simulink model "E33_VCU_simulink"  (R2014a)
settings: Solver=FixedStepDiscrete  StartTime=0.0  StopTime=10.0  FixedStep=0.0005  RelTol=1e-3
values from neighbouring files (symbols this model uses):
  Accu_FAN_Test = ecucoder_cal(Accu_FAN_Test)    [E33_VCU.m]
  Accu_FAN_threshold = ecucoder_cal(Accu_FAN_threshold)    [E33_VCU.m]
  APPS1_Voltage = ecucoder_cal(APPS1_Voltage)    [E33_VCU.m]
  APPS2_Voltage = ecucoder_cal(APPS2_Voltage)    [E33_VCU.m]
  APPS_Map = [0,1000]    [E33_VCU.m]
  APPS_threshold = ecucoder_cal(APPS_threshold)    [E33_VCU.m]
  Beep_Time = ecucoder_cal(Beep_Time)    [E33_VCU.m]
  BeeperTest = ecucoder_cal(BeeperTest)    [E33_VCU.m]
  BMSLedTest = ecucoder_cal(BMSLedTest)    [E33_VCU.m]
  BP_F_threshold = ecucoder_cal(BP_F_threshold)    [E33_VCU.m]
  BP_F_Voltage = ecucoder_cal(BP_F_Voltage)    [E33_VCU.m]
  BP_Map = [0,1000]    [E33_VCU.m]
  BP_R_Voltage = ecucoder_cal(BP_R_Voltage)    [E33_VCU.m]
  Brk_luminance = ecucoder_cal(Brk_luminance)    [E33_VCU.m]
  DCDC_Relay_Test = ecucoder_cal(DCDC_Relay_Test)    [E33_VCU.m]
  FactoryTestEnable = ecucoder_cal(FactoryTestEnable)    [E33_VCU.m]
  HardBrk_luminance = ecucoder_cal(HardBrk_luminance)    [E33_VCU.m]
  IMDLedTest = ecucoder_cal(IMDLedTest)    [E33_VCU.m]
  linear_FL_Map = ecucoder_cal(linear_FL_Map)    [E33_VCU.m]
  linear_FR_Map = ecucoder_cal(linear_FR_Map)    [E33_VCU.m]
  linear_Map = ecucoder_cal(linear_Map)    [E33_VCU.m]
  linear_RL_Map = ecucoder_cal(linear_RL_Map)    [E33_VCU.m]
  linear_RR_Map = ecucoder_cal(linear_RR_Map)    [E33_VCU.m]
  MaxPow = 40    [E33_VCU.m]
  MaxRPM = 5400    [E33_VCU.m]
  MaxRPMchangePerSec = ecucoder_cal(MaxRPMchangePerSec)    [E33_VCU.m]
  MaxTorqChangePerSec = ecucoder_cal(MaxTorqChangePerSec)    [E33_VCU.m]
  Motor_RPM_Map = (0:ceil(MaxRPM/100))*100    [E33_VCU.m]
  Pump_Test = ecucoder_cal(Pump_Test)    [E33_VCU.m]
  Pump_threshold = ecucoder_cal(Pump_threshold)    [E33_VCU.m]
  R2D_Light_Test = ecucoder_cal(R2D_Light_Test)    [E33_VCU.m]
  Radiator_FAN_Test = ecucoder_cal(Radiator_FAN_Test)    [E33_VCU.m]
  SCS_Error_5V = ecucoder_cal(SCS_Error_5V)    [E33_VCU.m]
  SCS_Error_GND = ecucoder_cal(SCS_Error_GND)    [E33_VCU.m]
  SPD_Coef = 1884/40    (= 47.1)    [E33_VCU.m]
  Tail_Light_Test = ecucoder_cal(Tail_Light_Test)    [E33_VCU.m]
  Tmanage_Map = [0,100]    [E33_VCU.m]
  Torq_percentage_Map = Motor_Torq_MAP/MaxTorq*1000    [E33_VCU.m]
libraries: simulink x164, ec55xxlib x44, dspswit3 x6
(part 1 of 5)
settings Model: Creator=lenovo  LastModifiedBy=lenovo
settings OptimizationCC: InlineParams=on  InlineInvariantSignals=on  RollThreshold=18  StateBitsets=on  DataBitsets=on  UseTempVars=on  ZeroExternalMemoryAtStartup=off  ZeroInternalMemoryAtStartup=off  EfficientFloat2IntCast=on  OptimizeModelRefInitCode=on  LifeSpan=1
settings DebuggingCC: InheritedTsInSrcMsg=none
settings HardwareCC: ProdLargestAtomicInteger=Long  ProdLargestAtomicFloat=Double  ProdIntDivRoundTo=Zero  ProdEndianess=BigEndian  ProdHWDeviceType=Freescale MPC5500
settings RTWCC: SystemTargetFile=ec55xx.tlc  MakeCommand=make_rtw optimized_fixed_point=1  GenerateMakefile=off  TemplateMakefile=ec55xx_lcc.tmf  PostCodeGenCommand=ec55xx_pst_s2(buildInfo)  Description=Target for EC55XX  GenerateReport=on  ProcessScript=ec55xx_make_rtw_hook  IncludeHyperlinkInReport=on  LaunchReport=on
settings CodeAppCC: IgnoreCustomStorageClasses=off
settings STFCustomTargetCC: ModelReferenceCompliant=off  ConcurrentExecutionCompliant=off  IncludeMdlTerminateFcn=off  GeneratePreprocessorConditionals=Use local settings  CombineOutputUpdateFcns=on  SuppressErrorStatus=on  ERTCustomFileBanners=on  SupportContinuousTime=off  SupportNonInlinedSFcns=off  MATLABClassNameForMDSCustomization=Simulink.SoftwareTarget.ERTCustomization  GRTInterface=off  SystemTargetFile=ec55xx.tlc
settings ERTTargetCC: GenerateSampleERTMain=off  ModelReferenceCompliant=off  IncludeMdlTerminateFcn=off  SuppressErrorStatus=on  GenerateASAP2=on  ERTSrcFileBannerTemplate=ec55xx_code_template.cgt  ERTHdrFileBannerTemplate=ec55xx_code_template.cgt  ERTDataSrcFileTemplate=ec55xx_code_template.cgt  ERTDataHdrFileTemplate=ec55xx_code_template.cgt  ERTCustomFileTemplate=ec55xx_file_process.tlc

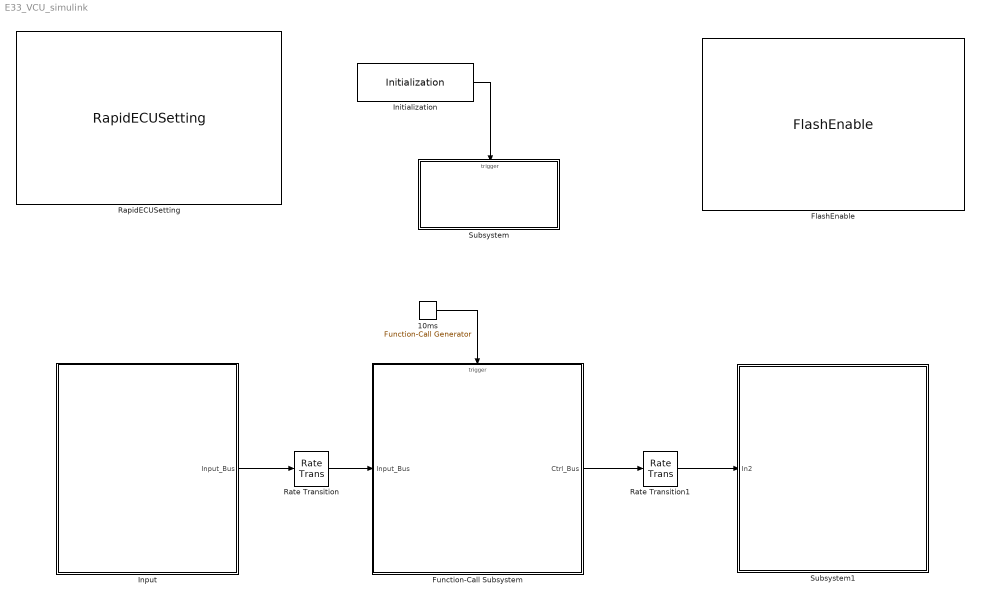
== system E33_VCU_simulink ==
  10ms : simulink/Ports & Subsystems/Function-Call Generator  sample_time=0.010  numberOfIterations=1
  FlashEnable : ec55xxlib/RapidECU_U2/10FlashManagement/FlashEnable  flashenable=on
  Function-Call Subsystem : Subsystem
  Initialization : ec55xxlib/RapidECU_U2/08MCUManagement/Initialization
  Input : Subsystem
  RapidECUSetting : ec55xxlib/RapidECU_U2/RapidECUSetting
      link override CAN: acmt=Extended(29-bit ID)  bcmt=Extended(29-bit ID)  apdf=1
      link override RTI: rtiperiod=0.0005
  Rate Transition : RateTransition
  Rate Transition1 : RateTransition
  Subsystem : Subsystem
  Subsystem1 : Subsystem
  wires:
  Initialization/1 -> Subsystem/Trigger
  Input/1(Input_Bus) -> Rate Transition/1
  Rate Transition/1 -> Function-Call Subsystem/1(Input_Bus)
  10ms/1 -> Function-Call Subsystem/Trigger
  Function-Call Subsystem/1(Ctrl_Bus) -> Rate Transition1/1
  Rate Transition1/1 -> Subsystem1/1(In2)

== system E33_VCU_simulink/Function-Call Subsystem ==
  Input_Bus : Inport
  function : TriggerPort  TriggerType=function-call
  Bus Creator : BusCreator  Inputs=2
  Bus Creator1 : BusCreator
  R2D_State : Subsystem
  Signal Conversion : SignalConversion
  Unit Delay : UnitDelay  SampleTime=-1
  Veh_Dynamic : Subsystem
  Warn : Subsystem
  Ctrl_Bus : Outport
  wires:
  Input_Bus/1 -> Bus Creator1/4, Bus Creator/2  "Input_Bus"
  Bus Creator1/1 -> Signal Conversion/1, Unit Delay/1  "Ctrl_Bus"
  Unit Delay/1 -> Bus Creator/1  "Ctrl_Bus_Delayed"
  Signal Conversion/1 -> Ctrl_Bus/1
  Bus Creator/1 -> R2D_State/1(In), Veh_Dynamic/1(Input_Bus), Warn/1(Warn_Msg)
  R2D_State/1(Out1) -> Bus Creator1/3  "R2D_State"
  Warn/1(Warn_level) -> Bus Creator1/1  "Warn"
  Veh_Dynamic/1(Out1) -> Bus Creator1/2  "Veh_Dynamic"

== system E33_VCU_simulink/Input ==
  Bus Creator : BusCreator  Inputs=6
  Input : Subsystem
  Input_Bus : Outport
  wires:
  Input/1("APP_Bus ") -> Bus Creator/1  "APP_Bus"
  Input/2("BP_Bus ") -> Bus Creator/2  "BP_Bus"
  Bus Creator/1 -> Input_Bus/1
  Input/3("Key_Bus ") -> Bus Creator/3  "Key_Bus"
  Input/4(Sensor_Bus) -> Bus Creator/4  "Sensor_Bus"
  Input/5(BMS_Bus) -> Bus Creator/5  "BMS_Bus"
  Input/6(MCU_Bus) -> Bus Creator/6  "MCU_Bus"

== system E33_VCU_simulink/Subsystem ==
  function : TriggerPort  TriggerType=function-call
  AfterRunSwitch : ec55xxlib/RapidECU_U2/09PowerManagement/AfterRunSwitch  sampletime=-1
  Constant : Constant  OutDataTypeStr=boolean
  PowerDriverSwitch : ec55xxlib/RapidECU_U2/04PowerDriverSwitch/PowerDriverSwitch  channel=99: O_MR_LS0A7  sampletime=-1
  wires:
  Constant/1 -> AfterRunSwitch/1, PowerDriverSwitch/1

== system E33_VCU_simulink/Subsystem1 ==
  In2 : Inport
  20ms : simulink/Ports & Subsystems/Function-Call Generator  sample_time=0.02  numberOfIterations=1
  20ms1 : simulink/Ports & Subsystems/Function-Call Generator  sample_time=0.02  numberOfIterations=1
  50ms{,1..3} (4 alike) : simulink/Ports & Subsystems/Function-Call Generator  sample_time=0.05  numberOfIterations=1
  DCDC_Ctrl : Subsystem
  MCUctrl : Subsystem  TreatAsAtomicUnit=on
  PanelCtrl : Subsystem  TreatAsAtomicUnit=on
  Rate Transition{1..6} (6 alike) : RateTransition
  TailLight : Subsystem  TreatAsAtomicUnit=on
  TmanageCtrl : Subsystem  TreatAsAtomicUnit=on
  VCUCAN : Subsystem
  wires:
  Rate Transition3/1 -> MCUctrl/1(In1)
  Rate Transition2/1 -> PanelCtrl/1(In1)
  50ms/1 -> PanelCtrl/Trigger
  20ms/1 -> MCUctrl/Trigger
  Rate Transition4/1 -> TailLight/1(In1)
  50ms1/1 -> TmanageCtrl/Trigger
  Rate Transition5/1 -> TmanageCtrl/1(In1)
  20ms1/1 -> TailLight/Trigger
  Rate Transition1/1 -> DCDC_Ctrl/1(In1)
  50ms2/1 -> DCDC_Ctrl/Trigger
  In2/1 -> Rate Transition3/1, Rate Transition6/1, Rate Transition1/1, Rate Transition5/1, Rate Transition4/1, Rate Transition2/1
  Rate Transition6/1 -> VCUCAN/1(In1)
  50ms3/1 -> VCUCAN/Trigger

== system E33_VCU_simulink/Function-Call Subsystem/R2D_State ==
  In : Inport
  Bus Creator1 : BusCreator  Inputs=3
  Bus Selector : BusSelector  OutputSignals=Input_Bus.Key_Bus.R2D_SW,Input_Bus.APP_Bus.APPS_Pos,Input_Bus.BP_Bus.BP_F_Pos,Input_Bus.MCU_Bus.MCU_Online,Input_Bus.MCU_Bus.MCU_Stat.MCU_IsReady
  Chart : Stateflow chart  RequirementInfo="{}  %GIDa_9082d276_9a80_43b5_a65a_81b478704c00"  TreatAsAtomicUnit=on
  Compare To Constant : simulink/Logic and Bit Operations/Compare To Constant  relop=<=  const=APPS_threshold  OutDataTypeStr=boolean
  Compare To Constant1 : simulink/Logic and Bit Operations/Compare To Constant  relop=>=  const=BP_F_threshold  OutDataTypeStr=boolean
  Constant : Constant  Value=Beep_Time
  Data Type Conversion{,1..3} (4 alike) : DataTypeConversion  OutDataTypeStr=boolean  RndMeth=Nearest
  Logical Operator : Logic  AllPortsSameDT=off  OutDataTypeStr=boolean
  Out1 : Outport
  wires:
  In/1 -> Bus Selector/1
  Bus Selector/2 -> Compare To Constant/1  "<APPS_Pos>"
  Bus Selector/3 -> Compare To Constant1/1  "<BP_F_Pos>"
  Bus Selector/4 -> Data Type Conversion/1  "<MCU_Online>"
  Bus Selector/5 -> Data Type Conversion1/1  "<MCU_IsReady>"
  Compare To Constant1/1 -> Data Type Conversion3/1
  Compare To Constant/1 -> Data Type Conversion2/1
  Chart/3(VehReady) -> Bus Creator1/3  "VehReady"
  Chart/2(VehStandby) -> Bus Creator1/2  "VehStandby"
  Chart/1(BeeperStOut) -> Bus Creator1/1  "BeeperOut"
  Bus Creator1/1 -> Out1/1
  Data Type Conversion/1 -> Logical Operator/1
  Data Type Conversion1/1 -> Logical Operator/2
  Logical Operator/1 -> Chart/4(MCU_Ready)  "MCU_Ready"
  Data Type Conversion2/1 -> Chart/2(APPS_OK)  "APPS_OK"
  Data Type Conversion3/1 -> Chart/3(BP_F_OK)  "BP_F_OK"
  Constant/1 -> Chart/5(Beep_Time)
  Bus Selector/1 -> Chart/1(R2D_SW)  "<R2D_SW>"

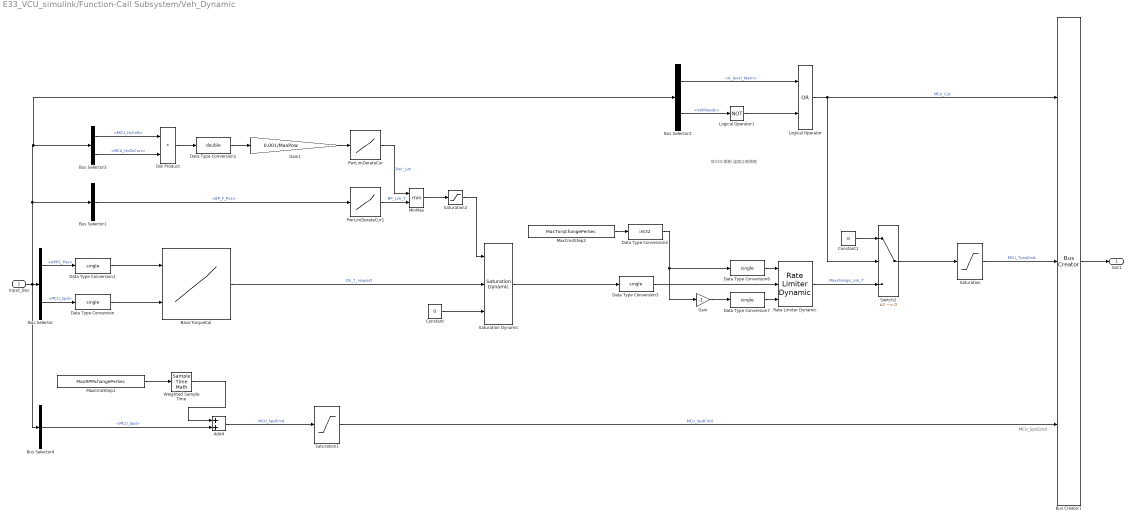
== system E33_VCU_simulink/Function-Call Subsystem/Veh_Dynamic ==
  note: 低SOC限制
      | 温度过高限制
  note: MCU_SpdCmd
  Input_Bus : Inport
  Add4 : Sum
  BasicTorqueCal : Lookup_n-D  BreakpointsForDimension1=[0,1000]  BreakpointsForDimension2=Motor_RPM_Map  Table=Torq_percentage_Map  TableDataTypeStr=Inherit: Inherit from 'Table data'  ExtrapMethod=Clip  InternalRulePriority=Speed  OutDataTypeStr=uint16  RndMeth=Simplest
  Bus Creator1 : BusCreator  Inputs=3
  Bus Selector : BusSelector  OutputSignals=Input_Bus.APP_Bus.APPS_Pos,Input_Bus.MCU_Bus.MCU_Stat.MCU_Spd
  Bus Selector1 : BusSelector  OutputSignals=Input_Bus.BP_Bus.BP_F_Pos
  Bus Selector2 : BusSelector  OutputSignals=Ctrl_Bus_Delayed.Warn.A_level_Warn,Ctrl_Bus_Delayed.R2D_State.VehReady
  Bus Selector3 : BusSelector  OutputSignals=Input_Bus.MCU_Bus.MCU_Power.MCU_HvVolt,Input_Bus.MCU_Bus.MCU_Power.MCU_HvDcCurr
  Bus Selector4 : BusSelector  OutputSignals=Input_Bus.MCU_Bus.MCU_Stat.MCU_Spd
  Constant : Constant  Value=0
  Constant1 : Constant  Value=0  OutDataTypeStr=uint16
  Data Type Conversion{,1,3,6..7} (5 alike) : DataTypeConversion  OutDataTypeStr=single
  Data Type Conversion2 : DataTypeConversion  OutDataTypeStr=double
  Data Type Conversion4 : DataTypeConversion  OutDataTypeStr=int32
  Dot Product : DotProduct  InputSameDT=on  OutDataTypeStr=Inherit: Inherit via internal rule
  Gain : Gain  Gain=-1
  Gain1 : Gain  Gain=0.001/MaxPow  OutDataTypeStr=single
  Logical Operator : Logic  Operator=OR  AllPortsSameDT=off  OutDataTypeStr=boolean
  Logical Operator1 : Logic  Operator=NOT  AllPortsSameDT=off  OutDataTypeStr=boolean
  MaxCmdStep1 : Constant  Value=MaxRPMchangePerSec  OutDataTypeStr=uint16
  MaxCmdStep2 : Constant  Value=MaxTorqChangePerSec  OutDataTypeStr=uint16
  MinMax : MinMax  Inputs=2
  PwrLimDerateCur : Lookup_n-D  NumberOfTableDimensions=1  BreakpointsForDimension1=[0.95,0.98,0.99]  BreakpointsForDimension1DataTypeStr=double  Table=[1000,500,0]  TableDataTypeStr=double  ExtrapMethod=Clip  InternalRulePriority=Speed  OutDataTypeStr=single  RndMeth=Simplest  InputSameDT=on
  PwrLimDerateCur1 : Lookup_n-D  NumberOfTableDimensions=1  BreakpointsForDimension1=[0,1000]  Table=[1000,0]  ExtrapMethod=Clip  InternalRulePriority=Speed  OutDataTypeStr=uint16  RndMeth=Simplest  InputSameDT=on
  Rate Limiter Dynamic : simulink/Discontinuities/Rate Limiter Dynamic
  Saturation : Saturate  UpperLimit=1000  LowerLimit=0
  Saturation Dynamic : simulink/Discontinuities/Saturation Dynamic  OutMin=[]  OutMax=[]  OutDataTypeStr=Inherit: Same as second input  OutDataType=fixdt(1, 16)  OutScaling=2^-10  DoSatur=off
  Saturation1 : Saturate  UpperLimit=MaxRPM  LowerLimit=-MaxRPM
  Saturation2 : Saturate  UpperLimit=1000  LowerLimit=0
  Switch2 : Switch  Criteria=u2 ~= 0
  Weighted Sample Time : SampleTimeMath  TsampMathOp=*
  Out1 : Outport
  wires:
  Input_Bus/1 -> Bus Selector4/1, Bus Selector2/1, Bus Selector3/1, Bus Selector1/1, Bus Selector/1
  Data Type Conversion/1 -> BasicTorqueCal/2
  Data Type Conversion1/1 -> BasicTorqueCal/1
  Bus Selector/1 -> Data Type Conversion1/1  "<APPS_Pos>"
  Bus Selector/2 -> Data Type Conversion/1  "<MCU_Spd>"
  Bus Selector1/1 -> PwrLimDerateCur1/1  "<BP_F_Pos>"
  Gain1/1 -> PwrLimDerateCur/1
  PwrLimDerateCur1/1 -> MinMax/2  "BP_Lim_T"
  PwrLimDerateCur/1 -> MinMax/1  "Pwr_Lim"
  MinMax/1 -> Saturation2/1
  Saturation2/1 -> Saturation Dynamic/1
  Dot Product/1 -> Data Type Conversion2/1
  Data Type Conversion2/1 -> Gain1/1
  Bus Selector3/1 -> Dot Product/1  "<MCU_HvVolt>"
  Bus Selector3/2 -> Dot Product/2  "<MCU_HvDcCurr>"
  BasicTorqueCal/1 -> Saturation Dynamic/2  "Dri_T_request"
  Constant/1 -> Saturation Dynamic/3
  Data Type Conversion4/1 -> Gain/1, Data Type Conversion6/1
  MaxCmdStep2/1 -> Data Type Conversion4/1
  Gain/1 -> Data Type Conversion7/1
  Data Type Conversion6/1 -> Rate Limiter Dynamic/1
  Data Type Conversion7/1 -> Rate Limiter Dynamic/3
  Data Type Conversion3/1 -> Rate Limiter Dynamic/2
  Logical Operator/1 -> Switch2/2, Bus Creator1/1  "MCU_Cut"
  Constant1/1 -> Switch2/1
  Saturation Dynamic/1 -> Data Type Conversion3/1
  Rate Limiter Dynamic/1 -> Switch2/3  "Maxchange_Lim_T"
  Switch2/1 -> Saturation/1
  Bus Selector4/1 -> Add4/2  "<MCU_Spd>"
  MaxCmdStep1/1 -> Weighted Sample Time/1
  Add4/1 -> Saturation1/1  "MCU_SpdCmd"
  Saturation/1 -> Bus Creator1/2  "MCU_TorqCmd"
  Saturation1/1 -> Bus Creator1/3  "MCU_SpdCmd"
  Bus Creator1/1 -> Out1/1
  Bus Selector2/1 -> Logical Operator/1  "<A_level_Warn>"
  Bus Selector2/2 -> Logical Operator1/1  "<VehReady>"
  Logical Operator1/1 -> Logical Operator/2
  Weighted Sample Time/1 -> Add4/1

== system E33_VCU_simulink/Function-Call Subsystem/Warn ==
  note: A级故障切断扭矩输出
      | B级故障显示告警信号
  Warn_Msg : Inport
  A_level_Warn : Subsystem
  B_level_Warn : Subsystem
  Bus Creator : BusCreator  Inputs=2
  Warn_level : Outport
  wires:
  Warn_Msg/1 -> B_level_Warn/1(In1), A_level_Warn/1(In1)
  A_level_Warn/1(A_level_Warn) -> Bus Creator/1  "A_level_Warn"
  B_level_Warn/1(B_level_Warn) -> Bus Creator/2  "B_level_Warn"
  Bus Creator/1 -> Warn_level/1

== system E33_VCU_simulink/Input/Input ==
  100ms : simulink/Ports & Subsystems/Function-Call Generator  sample_time=0.1  numberOfIterations=1
  10ms{,1..4} (5 alike) : simulink/Ports & Subsystems/Function-Call Generator  sample_time=0.010  numberOfIterations=1
  50ms : simulink/Ports & Subsystems/Function-Call Generator  sample_time=0.050  numberOfIterations=1
  APPS : Subsystem
  BMS_CAN_Receive : Subsystem  TreatAsAtomicUnit=on
  Bpressure : Subsystem
  Bus Creator : BusCreator
  Bus Creator1 : BusCreator
  Bus Creator2 : BusCreator  Inputs=1
  Bus Creator3 : BusCreator  Inputs=5
  Bus Creator4 : BusCreator  Inputs=5
  Bus Creator5 : BusCreator  Inputs=3
  Keys : Subsystem
  MCU_CAN_Receive : Subsystem
  Self_inspection : Subsystem
  Sensor : Subsystem
  "APP_Bus " : Outport
  "BP_Bus " : Outport  Port=2
  "Key_Bus " : Outport  Port=3
  Sensor_Bus : Outport  Port=4
  BMS_Bus : Outport  Port=5
  MCU_Bus : Outport  Port=6
  wires:
  10ms/1 -> APPS/Trigger
  10ms1/1 -> Bpressure/Trigger
  APPS/2(APPS_Unreliable) -> Bus Creator/2  "APPS_Unreliable"
  APPS/1(APPS_Pos) -> Bus Creator/1  "APPS_Pos"
  Bus Creator/1 -> "APP_Bus "/1
  Bus Creator1/1 -> "BP_Bus "/1
  50ms/1 -> Self_inspection/Trigger
  Bus Creator2/1 -> "Key_Bus "/1
  Keys/1(R2D_SW) -> Bus Creator2/1  "R2D_SW"
  10ms2/1 -> Keys/Trigger
  10ms3/1 -> Sensor/Trigger
  Sensor/1(Linear_RR) -> Bus Creator3/1  "Linear_RR"
  Sensor/3(Linear_RL) -> Bus Creator3/3  "Linear_RL"
  Sensor/2(Linear_FR) -> Bus Creator3/2  "Linear_FR"
  Sensor/4(Linear_FL) -> Bus Creator3/4  "Linear_FL"
  Sensor/5(Wheel_Angle) -> Bus Creator3/5  "Wheel_Angle"
  Bus Creator3/1 -> Sensor_Bus/1
  10ms4/1 -> MCU_CAN_Receive/Trigger
  100ms/1 -> BMS_CAN_Receive/Trigger
  BMS_CAN_Receive/2(BMS_INFO) -> Bus Creator4/2  "BMS_Info"
  Bus Creator4/1 -> BMS_Bus/1
  BMS_CAN_Receive/1(BMS_Online) -> Bus Creator4/1  "BMS_Online"
  BMS_CAN_Receive/3(BMS_ALM) -> Bus Creator4/3  "BMS_Alarm"
  BMS_CAN_Receive/4(BMS_MAXT) -> Bus Creator4/4  "BMS_MAXT"
  MCU_CAN_Receive/3(MCU_Power) -> Bus Creator5/3  "MCU_Power"
  MCU_CAN_Receive/2(MCU_Stat) -> Bus Creator5/2  "MCU_Stat"
  MCU_CAN_Receive/1(MCU_Online) -> Bus Creator5/1  "MCU_Online"
  Bus Creator5/1 -> MCU_Bus/1
  BMS_CAN_Receive/5(BMS_MAXV) -> Bus Creator4/5  "BMS_MAXV"
  APPS/3(APPS1_Disconnect) -> Bus Creator/3  "APPS1_Disconnect"
  APPS/4(APPS2_Disconnect) -> Bus Creator/4  "APPS2_Disconnect"
  Bpressure/3(BP_F_Disconnect) -> Bus Creator1/3  "BP_F_Disconnect"
  Bpressure/4(BP_R_Disconnect) -> Bus Creator1/4  "BP_R_Disconnect"
  Bpressure/1(BP_F_Pos) -> Bus Creator1/1  "BP_F_Pos"
  Bpressure/2(BP_R_Pos) -> Bus Creator1/2  "BP_R_Pos"

== system E33_VCU_simulink/Subsystem1/DCDC_Ctrl ==
  In1 : Inport
  function : TriggerPort  TriggerType=function-call
  Bus Selector3 : BusSelector  OutputSignals=Input_Bus.BMS_Bus.BMS_Info.BMS_Stat,Input_Bus.BMS_Bus.BMS_Online
  Compare To Constant1 : simulink/Logic and Bit Operations/Compare To Constant  relop===  const=5  OutDataTypeStr=boolean
  Constant4 : Constant  Value=FactoryTestEnable  OutDataTypeStr=Inherit: Inherit via back propagation
  Constant5 : Constant  Value=DCDC_Relay_Test  OutDataTypeStr=Inherit: Inherit via back propagation
  DCDC_Ctrl : Stateflow chart  TreatAsAtomicUnit=on
  DCDC_MR_CTRL : ec55xxlib/RapidECU_U2/04PowerDriverSwitch/PowerDriverSwitch  channel=60: O_PWM3_LS1A8  sampletime=-1
  Data Type Conversion3 : DataTypeConversion  OutDataTypeStr=boolean
  Logical Operator1 : Logic  AllPortsSameDT=off  OutDataTypeStr=boolean
  Switch1 : Switch  Criteria=u2 ~= 0
  wires:
  In1/1 -> Bus Selector3/1
  Logical Operator1/1 -> DCDC_Ctrl/1(HV_ON)
  Bus Selector3/2 -> Logical Operator1/2  "<BMS_Online>"
  Data Type Conversion3/1 -> Switch1/3  "DCDC_ON"
  Bus Selector3/1 -> Compare To Constant1/1  "<BMS_Stat>"
  Compare To Constant1/1 -> Logical Operator1/1
  Constant5/1 -> Switch1/1
  DCDC_Ctrl/1(DCDC_ON) -> Data Type Conversion3/1
  Switch1/1 -> DCDC_MR_CTRL/1  "DCDC_MR"
  Constant4/1 -> Switch1/2

== system E33_VCU_simulink/Subsystem1/MCUctrl ==
  In1 : Inport
  function : TriggerPort  TriggerType=function-call
  Bus Selector : BusSelector  OutputSignals=Veh_Dynamic.MCU_Cut,Veh_Dynamic.MCU_TorqCmd,Veh_Dynamic.MCU_SpdCmd
  Bus Selector1 : BusSelector  OutputSignals=Input_Bus.MCU_Bus.MCU_Online
  Constant : Constant
  Constant{1..5,8..9} (7 alike) : Constant  Value=0
  Constant10 : Constant
  Constant6 : Constant  Value=0  OutDataTypeStr=uint8
  Constant7 : Constant  Value=2
  Data Type Conversion{1..9} (9 alike) : DataTypeConversion  OutDataTypeStr=uint16
  Data Type Conversion10 : DataTypeConversion  OutDataTypeStr=int32
  Data Type Conversion11 : DataTypeConversion  OutDataTypeStr=int32
  In2 : InportShadow
  MCU_CMD_CAN_Tx : Subsystem  TreatAsAtomicUnit=on
  Switch1 : Switch  Criteria=u2 ~= 0
  Switch2 : Switch  Criteria=u2 ~= 0
  Terminator1 : Terminator
  VCU_MCU_CMD : Subsystem
  wires:
  In1/1 -> Bus Selector/1
  Constant/1 -> Data Type Conversion2/1
  Constant7/1 -> Switch1/3
  Constant1/1 -> Data Type Conversion5/1
  Constant2/1 -> Data Type Conversion6/1
  Constant3/1 -> Data Type Conversion7/1
  Constant4/1 -> Data Type Conversion9/1
  Switch2/1 -> Data Type Conversion8/1
  Bus Selector/2 -> Data Type Conversion10/1  "<MCU_TorqCmd>"
  Bus Selector/3 -> Data Type Conversion11/1  "<MCU_SpdCmd>"
  Bus Selector/1 -> Switch1/2, Switch2/2  "<MCU_Cut>"
  Constant6/1 -> Data Type Conversion1/1
  Data Type Conversion4/1 -> VCU_MCU_CMD/4(MCU_IsMcuNOTActive_in)
  Data Type Conversion1/1 -> VCU_MCU_CMD/1(MCU_HV_Voltage_in)
  Data Type Conversion2/1 -> VCU_MCU_CMD/2(MCU_IsPosRelayAct_in)
  Data Type Conversion3/1 -> VCU_MCU_CMD/3(MCU_GEAR_CMD_in)
  Data Type Conversion5/1 -> VCU_MCU_CMD/5(MCU_IsZeroLocMode_in)
  Data Type Conversion6/1 -> VCU_MCU_CMD/6(MCU_IsBrakeMode_in)
  Data Type Conversion7/1 -> VCU_MCU_CMD/7(MCU_IsSpdMode_in)
  Data Type Conversion8/1 -> VCU_MCU_CMD/8(MCU_IsTorqMode_in)
  Data Type Conversion9/1 -> VCU_MCU_CMD/9(MCU_IsFreeMode_in)
  Data Type Conversion10/1 -> VCU_MCU_CMD/10(MCU_TORQ_CMD_in)
  Data Type Conversion11/1 -> VCU_MCU_CMD/11(MCU_SPD_CMD_in)
  MCU_CMD_CAN_Tx/1(CAN_OK) -> Terminator1/1
  Switch1/1 -> Data Type Conversion3/1
  Constant8/1 -> Switch1/1
  Constant9/1 -> Data Type Conversion4/1
  Constant5/1 -> Switch2/1
  Constant10/1 -> Switch2/3
  VCU_MCU_CMD/1(output) -> MCU_CMD_CAN_Tx/1(Msg)
  In2/1 -> Bus Selector1/1
  Bus Selector1/1 -> MCU_CMD_CAN_Tx/Enable  "<MCU_Online>"

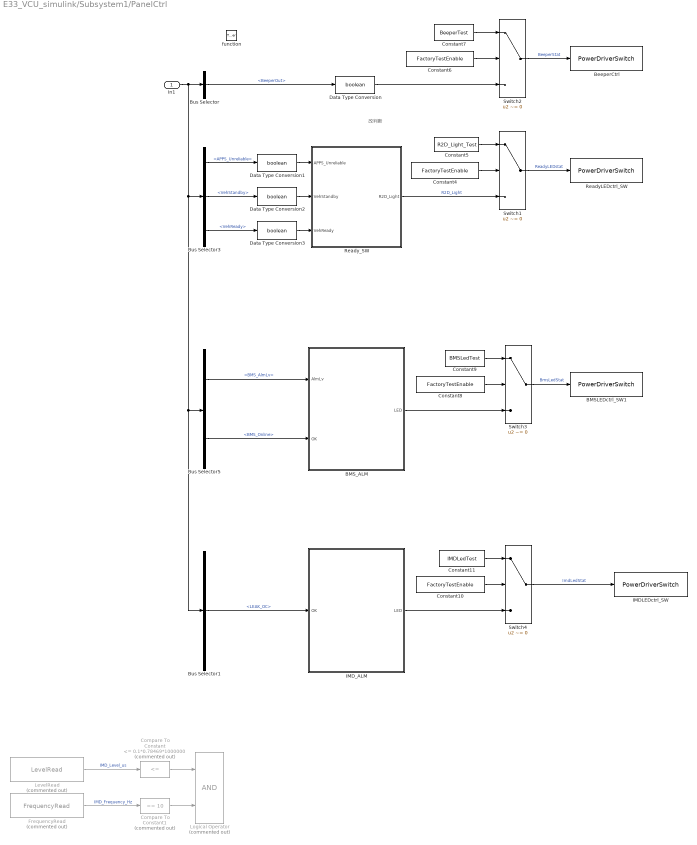
== system E33_VCU_simulink/Subsystem1/PanelCtrl ==
  note: 改判断
  In1 : Inport
  function : TriggerPort  TriggerType=function-call
  BMSLEDctrl_SW1 : ec55xxlib/RapidECU_U2/04PowerDriverSwitch/PowerDriverSwitch  channel=63: O_SW1_LS0A7  sampletime=-1
  BMS_ALM : Stateflow chart  TreatAsAtomicUnit=on
  BeeperCtrl : ec55xxlib/RapidECU_U2/04PowerDriverSwitch/PowerDriverSwitch  channel=79: O_SW3_LS0A7  sampletime=-1
  Bus Selector : BusSelector  OutputSignals=R2D_State.BeeperOut
  Bus Selector1 : BusSelector  OutputSignals=Input_Bus.BMS_Bus.BMS_Alarm.LEAK_OC
  Bus Selector3 : BusSelector  OutputSignals=Input_Bus.APP_Bus.APPS_Unreliable,R2D_State.VehStandby,R2D_State.VehReady
  Bus Selector5 : BusSelector  OutputSignals=Input_Bus.BMS_Bus.BMS_Info.BMS_AlmLv,Input_Bus.BMS_Bus.BMS_Online
  Compare To Constant : simulink/Logic and Bit Operations/Compare To Constant  Commented=on  relop=<=  const=0.1*0.78469*1000000  OutDataTypeStr=boolean
  Compare To Constant1 : simulink/Logic and Bit Operations/Compare To Constant  Commented=on  relop===  const=10  OutDataTypeStr=boolean
  Constant{4,6,8,10} (4 alike) : Constant  Value=FactoryTestEnable  OutDataTypeStr=Inherit: Inherit via back propagation
  Constant11 : Constant  Value=IMDLedTest  OutDataTypeStr=Inherit: Inherit via back propagation
  Constant5 : Constant  Value=R2D_Light_Test  OutDataTypeStr=Inherit: Inherit via back propagation
  Constant7 : Constant  Value=BeeperTest  OutDataTypeStr=Inherit: Inherit via back propagation
  Constant9 : Constant  Value=BMSLedTest  OutDataTypeStr=Inherit: Inherit via back propagation
  Data Type Conversion{,1..3} (4 alike) : DataTypeConversion  OutDataTypeStr=boolean
  FrequencyRead : ec55xxlib/RapidECU_U2/03FrequencyInput/FrequencyRead  Commented=on  channel=37: I_HALL1  sampletime=-1
  IMDLEDctrl_SW : ec55xxlib/RapidECU_U2/04PowerDriverSwitch/PowerDriverSwitch  channel=78: O_SW2_LS0A7  sampletime=-1
  IMD_ALM : Stateflow chart  TreatAsAtomicUnit=on
  LevelRead : ec55xxlib/RapidECU_U2/03FrequencyInput/LevelRead  Commented=on  channel=37: I_HALL1  activelevel=Active High  sampletime=-1
  Logical Operator : Logic  Commented=on  AllPortsSameDT=off  OutDataTypeStr=boolean
  ReadyLEDctrl_SW : ec55xxlib/RapidECU_U2/04PowerDriverSwitch/PowerDriverSwitch  channel=58: O_PWM1_LS1A8  sampletime=-1
  Ready_SW : Stateflow chart  TreatAsAtomicUnit=on
  Switch{1..4} (4 alike) : Switch  Criteria=u2 ~= 0
  wires:
  Bus Selector/1 -> Data Type Conversion/1  "<BeeperOut>"
  In1/1 -> Bus Selector1/1, Bus Selector5/1, Bus Selector3/1, Bus Selector/1
  Ready_SW/1(R2D_Light) -> Switch1/3  "R2D_Light"
  Constant4/1 -> Switch1/2
  Constant5/1 -> Switch1/1
  Switch1/1 -> ReadyLEDctrl_SW/1  "ReadyLEDstat"
  Data Type Conversion/1 -> Switch2/3
  Constant6/1 -> Switch2/2
  Constant7/1 -> Switch2/1
  Switch2/1 -> BeeperCtrl/1  "BeeperStat"
  BMS_ALM/1(LED) -> Switch3/3
  Constant8/1 -> Switch3/2
  Constant9/1 -> Switch3/1
  Switch3/1 -> BMSLEDctrl_SW1/1  "BmsLedStat"
  Constant10/1 -> Switch4/2
  Constant11/1 -> Switch4/1
  Bus Selector5/1 -> BMS_ALM/1(AlmLv)  "<BMS_AlmLv>"
  Bus Selector5/2 -> BMS_ALM/2(OK)  "<BMS_Online>"
  Bus Selector3/1 -> Data Type Conversion1/1  "<APPS_Unreliable>"
  Bus Selector3/2 -> Data Type Conversion2/1  "<VehStandby>"
  Bus Selector3/3 -> Data Type Conversion3/1  "<VehReady>"
  Data Type Conversion1/1 -> Ready_SW/1(APPS_Unreliable)
  Data Type Conversion2/1 -> Ready_SW/2(VehStandby)
  Data Type Conversion3/1 -> Ready_SW/3(VehReady)
  FrequencyRead/1 -> Compare To Constant1/1  "IMD_Frequency_Hz"
  LevelRead/1 -> Compare To Constant/1  "IMD_Level_us"
  Compare To Constant/1 -> Logical Operator/1
  Compare To Constant1/1 -> Logical Operator/2
  Bus Selector1/1 -> IMD_ALM/1(OK)  "<LEAK_OC>"
  IMD_ALM/1(LED) -> Switch4/3
  Switch4/1 -> IMDLEDctrl_SW/1  "ImdLedStat"

== system E33_VCU_simulink/Subsystem1/TailLight ==
  In1 : Inport
  function : TriggerPort  TriggerType=function-call
  Bus Selector1 : BusSelector  OutputSignals=Input_Bus.BP_Bus.BP_F_Pos
  Compare To Constant : simulink/Logic and Bit Operations/Compare To Constant  relop=>=  const=80  OutDataTypeStr=boolean
  Compare To Constant1 : simulink/Logic and Bit Operations/Compare To Constant  relop=>=  const=950  OutDataTypeStr=boolean
  Constant : Constant  Value=5000  OutDataTypeStr=uint32
  Constant1 : Constant  Value=Brk_luminance
  Constant2 : Constant  Value=HardBrk_luminance
  Constant5 : Constant  Value=Tail_Light_Test  OutDataTypeStr=uint32
  Constant8 : Constant  Value=FactoryTestEnable  OutDataTypeStr=Inherit: Inherit via back propagation
  Data Type Conversion1 : DataTypeConversion  OutDataTypeStr=uint32
  Gain : Gain  Gain=50
  LED : Stateflow chart  TreatAsAtomicUnit=on
  Switch1 : Switch  Criteria=u2 ~= 0
  TailLightctrl : ec55xxlib/RapidECU_U2/06PowerDriverPWM/PowerDriverPWM  channel=61: O_PWM4_LS1A8  sampletime=-1
  wires:
  Constant/1 -> TailLightctrl/1
  Data Type Conversion1/1 -> TailLightctrl/2  "TailLightOnTime"
  In1/1 -> Bus Selector1/1
  Gain/1 -> Data Type Conversion1/1
  LED/1(LEDDutyCyc) -> Switch1/3
  Switch1/1 -> Gain/1
  Bus Selector1/1 -> Compare To Constant1/1, Compare To Constant/1  "<BP_F_Pos>"
  Compare To Constant1/1 -> LED/2(IsHardBrk)
  Compare To Constant/1 -> LED/1(IsBrk)
  Constant5/1 -> Switch1/1
  Constant8/1 -> Switch1/2
  Constant1/1 -> LED/3(Brk_luminance)
  Constant2/1 -> LED/4(HardBrk_luminance)

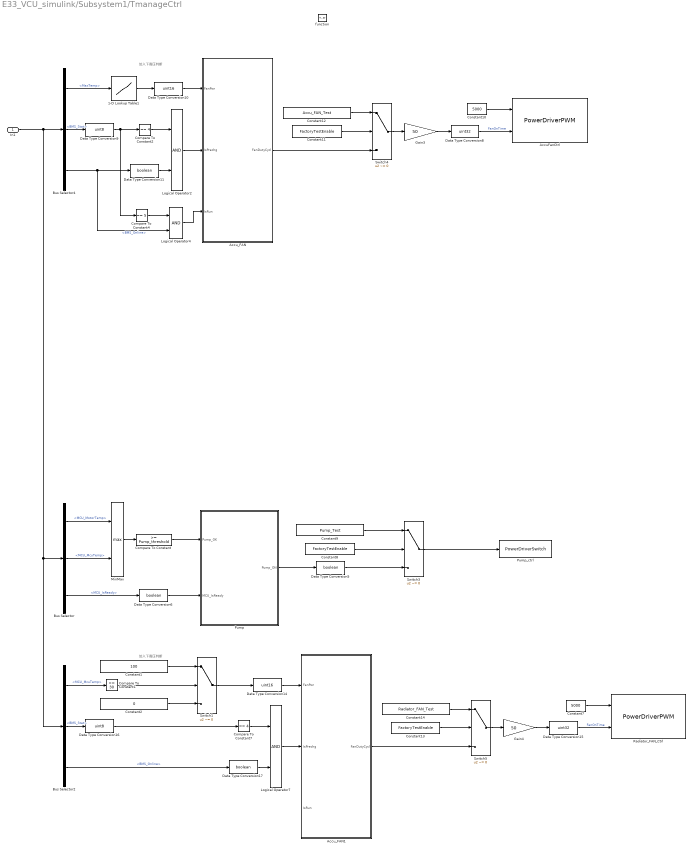
== system E33_VCU_simulink/Subsystem1/TmanageCtrl ==
  note: 加入下高压判断
  note: 加入下高压判断
  In1 : Inport
  function : TriggerPort  TriggerType=function-call
  1-D Lookup Table1 : Lookup_n-D  NumberOfTableDimensions=1  BreakpointsForDimension1=Accu_FAN_threshold  Table=Tmanage_Map  ExtrapMethod=Clip  InternalRulePriority=Speed  RndMeth=Simplest  InputSameDT=on
  AccuFanCtrl : ec55xxlib/RapidECU_U2/06PowerDriverPWM/PowerDriverPWM  channel=117: O_PWM11_HS2A9  sampletime=-1
  Accu_FAN : Stateflow chart  TreatAsAtomicUnit=on
  Accu_FAN1 : Stateflow chart  TreatAsAtomicUnit=on
  Bus Selector : BusSelector  OutputSignals=Input_Bus.MCU_Bus.MCU_Power.MCU_MotorTemp,Input_Bus.MCU_Bus.MCU_Power.MCU_McuTemp,Input_Bus.MCU_Bus.MCU_Stat.MCU_IsReady
  Bus Selector2 : BusSelector  OutputSignals=Input_Bus.MCU_Bus.MCU_Power.MCU_McuTemp,Input_Bus.BMS_Bus.BMS_Info.BMS_Stat,Input_Bus.BMS_Bus.BMS_Online
  Bus Selector4 : BusSelector  OutputSignals=Input_Bus.BMS_Bus.BMS_MAXT.MaxTemp,Input_Bus.BMS_Bus.BMS_Info.BMS_Stat,Input_Bus.BMS_Bus.BMS_Online
  Compare To Constant : simulink/Logic and Bit Operations/Compare To Constant  relop=>=  const=Pump_threshold  OutDataTypeStr=boolean
  Compare To Constant1 : simulink/Logic and Bit Operations/Compare To Constant  relop=>=  const=30  OutDataTypeStr=boolean
  Compare To Constant2 : simulink/Logic and Bit Operations/Compare To Constant  relop===  const=4  OutDataTypeStr=boolean
  Compare To Constant4 : simulink/Logic and Bit Operations/Compare To Constant  relop===  const=5  OutDataTypeStr=boolean
  Compare To Constant7 : simulink/Logic and Bit Operations/Compare To Constant  relop===  const=4  OutDataTypeStr=boolean
  Constant1 : Constant  Value=100  OutDataTypeStr=uint32
  Constant10 : Constant  Value=5000  OutDataTypeStr=uint32
  Constant11 : Constant  Value=FactoryTestEnable  OutDataTypeStr=Inherit: Inherit via back propagation
  Constant12 : Constant  Value=Accu_FAN_Test  OutDataTypeStr=uint32
  Constant13 : Constant  Value=FactoryTestEnable  OutDataTypeStr=Inherit: Inherit via back propagation
  Constant14 : Constant  Value=Radiator_FAN_Test  OutDataTypeStr=uint32
  Constant2 : Constant  Value=0  OutDataTypeStr=uint32
  Constant7 : Constant  Value=5000  OutDataTypeStr=uint32
  Constant8 : Constant  Value=FactoryTestEnable  OutDataTypeStr=Inherit: Inherit via back propagation
  Constant9 : Constant  Value=Pump_Test  OutDataTypeStr=Inherit: Inherit via back propagation
  Data Type Conversion10 : DataTypeConversion  OutDataTypeStr=uint16
  Data Type Conversion{5..6,11,17} (4 alike) : DataTypeConversion  OutDataTypeStr=boolean
  Data Type Conversion14 : DataTypeConversion  OutDataTypeStr=uint16
  Data Type Conversion15 : DataTypeConversion  OutDataTypeStr=uint32
  Data Type Conversion16 : DataTypeConversion  OutDataTypeStr=uint8
  Data Type Conversion8 : DataTypeConversion  OutDataTypeStr=uint32
  Data Type Conversion9 : DataTypeConversion  OutDataTypeStr=uint8
  Gain3 : Gain  Gain=50
  Gain4 : Gain  Gain=50
  Logical Operator2 : Logic  AllPortsSameDT=off  OutDataTypeStr=boolean
  Logical Operator4 : Logic  AllPortsSameDT=off  OutDataTypeStr=boolean
  Logical Operator7 : Logic  AllPortsSameDT=off  OutDataTypeStr=boolean
  MinMax : MinMax  Function=max  Inputs=2
  Pump : Stateflow chart  TreatAsAtomicUnit=on
  Pump_ctrl : ec55xxlib/RapidECU_U2/04PowerDriverSwitch/PowerDriverSwitch  channel=59: O_PWM2_LS1A8  sampletime=-1
  Radiator_FAN_Ctrl : ec55xxlib/RapidECU_U2/06PowerDriverPWM/PowerDriverPWM  channel=115: O_PWM10_HS2A9  sampletime=-1
  Switch{1,3..5} (4 alike) : Switch  Criteria=u2 ~= 0
  wires:
  Constant10/1 -> AccuFanCtrl/1
  Data Type Conversion8/1 -> AccuFanCtrl/2  "FanOnTime"
  Gain3/1 -> Data Type Conversion8/1
  Accu_FAN/1(FanDutyCycl) -> Switch4/3
  Constant11/1 -> Switch4/2
  Constant12/1 -> Switch4/1
  Switch4/1 -> Gain3/1
  Data Type Conversion9/1 -> Compare To Constant2/1, Compare To Constant4/1
  Compare To Constant2/1 -> Logical Operator2/1
  Bus Selector4/1 -> 1-D Lookup Table1/1  "<MaxTemp>"
  1-D Lookup Table1/1 -> Data Type Conversion10/1
  Data Type Conversion10/1 -> Accu_FAN/1(FanPwr)
  Logical Operator2/1 -> Accu_FAN/2(IsPrechg)
  Data Type Conversion11/1 -> Logical Operator2/2
  Bus Selector4/2 -> Data Type Conversion9/1  "<BMS_Stat>"
  Bus Selector4/3 -> Logical Operator4/2, Data Type Conversion11/1  "<BMS_Online>"
  Compare To Constant4/1 -> Logical Operator4/1
  Logical Operator4/1 -> Accu_FAN/3(IsRun)
  Constant7/1 -> Radiator_FAN_Ctrl/1
  Data Type Conversion15/1 -> Radiator_FAN_Ctrl/2  "FanOnTime"
  Gain4/1 -> Data Type Conversion15/1
  Accu_FAN1/1(FanDutyCycl) -> Switch5/3
  Constant13/1 -> Switch5/2
  Constant14/1 -> Switch5/1
  Switch5/1 -> Gain4/1
  Data Type Conversion16/1 -> Compare To Constant7/1
  Compare To Constant7/1 -> Logical Operator7/1
  Bus Selector2/1 -> Compare To Constant1/1  "<MCU_McuTemp>"
  Switch1/1 -> Data Type Conversion14/1
  Data Type Conversion14/1 -> Accu_FAN1/1(FanPwr)
  Logical Operator7/1 -> Accu_FAN1/2(IsPrechg)
  Data Type Conversion17/1 -> Logical Operator7/2
  Bus Selector2/2 -> Data Type Conversion16/1  "<BMS_Stat>"
  Bus Selector2/3 -> Data Type Conversion17/1  "<BMS_Online>"
  Constant8/1 -> Switch3/2
  Bus Selector/2 -> MinMax/2  "<MCU_McuTemp>"
  Bus Selector/1 -> MinMax/1  "<MCU_MotorTemp>"
  MinMax/1 -> Compare To Constant/1
  In1/1 -> Bus Selector/1, Bus Selector2/1, Bus Selector4/1
  Bus Selector/3 -> Data Type Conversion6/1  "<MCU_IsReady>"
  Compare To Constant/1 -> Pump/1(Pump_OK)
  Pump/1(Pump_ON) -> Data Type Conversion5/1
  Data Type Conversion5/1 -> Switch3/3
  Constant9/1 -> Switch3/1
  Data Type Conversion6/1 -> Pump/2(MCU_IsReady)
  Switch3/1 -> Pump_ctrl/1
  Constant1/1 -> Switch1/1
  Compare To Constant1/1 -> Switch1/2
  Constant2/1 -> Switch1/3

== system E33_VCU_simulink/Subsystem1/VCUCAN ==
  In1 : Inport
  function : TriggerPort  TriggerType=function-call
  Bus Selector3 : BusSelector  OutputSignals=Input_Bus.Sensor_Bus.Linear_RR,Input_Bus.Sensor_Bus.Linear_FR,Input_Bus.Sensor_Bus.Linear_RL,Input_Bus.Sensor_Bus.Linear_FL,Input_Bus.Sensor_Bus.Wheel_Angle
  CANTransmit : ec55xxlib/RapidECU_U2/07CANCommucation/CANTransmit  canmodule=A  canbuffer=8  canmessageid=hex2dec('17000000')  canmessagetype=Extended(29-bit ID)  datalength=8  sampletime=-1
  Terminator1 : Terminator
  VCU_Panel : Subsystem
  wires:
  In1/1 -> Bus Selector3/1
  CANTransmit/1 -> Terminator1/1
  Bus Selector3/1 -> VCU_Panel/2(Linear_RR_in)  "<Linear_RR>"
  Bus Selector3/2 -> VCU_Panel/3(Linear_FR_in)  "<Linear_FR>"
  Bus Selector3/3 -> VCU_Panel/4(Linear_RL_in)  "<Linear_RL>"
  Bus Selector3/4 -> VCU_Panel/5(Linear_FL_in)  "<Linear_FL>"
  Bus Selector3/5 -> VCU_Panel/1(Wheel_Angle_in)  "<Wheel_Angle>"
  VCU_Panel/1(output) -> CANTransmit/1

== system E33_VCU_simulink/Function-Call Subsystem/Warn/A_level_Warn ==
  In1 : Inport
  Bus Selector : BusSelector  OutputSignals=Input_Bus.MCU_Bus.MCU_Online,Input_Bus.APP_Bus.APPS_Unreliable,Input_Bus.APP_Bus.APPS1_Disconnect,Input_Bus.APP_Bus.APPS2_Disconnect,Input_Bus.BP_Bus.BP_F_Disconnect,Input_Bus.BP_Bus.BP_R_Disconnect
  Compare To Constant : simulink/Logic and Bit Operations/Compare To Constant  relop===  const=1  OutDataTypeStr=boolean
  Compare To Constant1 : simulink/Logic and Bit Operations/Compare To Constant  relop===  const=1  OutDataTypeStr=boolean
  Compare To Constant2 : simulink/Logic and Bit Operations/Compare To Constant  relop===  const=1  OutDataTypeStr=boolean
  Compare To Constant5 : simulink/Logic and Bit Operations/Compare To Constant  relop=~=  const=1  OutDataTypeStr=boolean
  Data Type Conversion{,1..2,5} (4 alike) : DataTypeConversion  OutDataTypeStr=boolean
  Logical Operator : Logic  Operator=OR  Inputs=1  IconShape=distinctive  AllPortsSameDT=off  OutDataTypeStr=boolean
  Mux : Mux  Inputs=6
  A_level_Warn : Outport
  wires:
  In1/1 -> Bus Selector/1
  Data Type Conversion/1 -> Compare To Constant/1
  Data Type Conversion1/1 -> Compare To Constant1/1
  Data Type Conversion2/1 -> Compare To Constant2/1
  Bus Selector/1 -> Data Type Conversion5/1  "<MCU_Online>"
  Data Type Conversion5/1 -> Compare To Constant5/1
  Logical Operator/1 -> A_level_Warn/1
  Mux/1 -> Logical Operator/1
  Bus Selector/2 -> Data Type Conversion/1  "<APPS_Unreliable>"
  Bus Selector/3 -> Data Type Conversion1/1  "<APPS1_Disconnect>"
  Bus Selector/4 -> Data Type Conversion2/1  "<APPS2_Disconnect>"
  Compare To Constant/1 -> Mux/2  "Bad_APPAlm"
  Compare To Constant1/1 -> Mux/3  "BadApp1Alm"
  Compare To Constant2/1 -> Mux/4  "BadApp2Alm"
  Compare To Constant5/1 -> Mux/1  "BadMcuAlm"

== system E33_VCU_simulink/Function-Call Subsystem/Warn/B_level_Warn ==
  In1 : Inport
  Bus Selector : BusSelector  OutputSignals=Input_Bus.BMS_Bus.BMS_Info.BMS_AlmLv,Input_Bus.BMS_Bus.BMS_Online
  Compare To Constant1 : simulink/Logic and Bit Operations/Compare To Constant  relop=~=  const=0  OutDataTypeStr=boolean
  Compare To Constant2 : simulink/Logic and Bit Operations/Compare To Constant  relop===  const=0  OutDataTypeStr=boolean
  Data Type Conversion1 : DataTypeConversion  OutDataTypeStr=uint8  RndMeth=Nearest
  Data Type Conversion2 : DataTypeConversion  OutDataTypeStr=boolean
  Logical Operator : Logic  Operator=OR  Inputs=1  IconShape=distinctive  AllPortsSameDT=off  OutDataTypeStr=boolean
  Mux : Mux  Inputs=2
  B_level_Warn : Outport
  wires:
  In1/1 -> Bus Selector/1
  Data Type Conversion1/1 -> Compare To Constant1/1
  Data Type Conversion2/1 -> Compare To Constant2/1
  Compare To Constant1/1 -> Mux/1
  Compare To Constant2/1 -> Mux/2
  Logical Operator/1 -> B_level_Warn/1
  Bus Selector/2 -> Data Type Conversion2/1  "<BMS_Online>"
  Bus Selector/1 -> Data Type Conversion1/1  "<BMS_AlmLv>"
  Mux/1 -> Logical Operator/1

== system E33_VCU_simulink/Input/Input/APPS ==
  function : TriggerPort  TriggerType=function-call
  1-D Lookup Table : Lookup_n-D  NumberOfTableDimensions=1  BreakpointsForDimension1=APPS1_Voltage  Table=APPS_Map  ExtrapMethod=Clip  InternalRulePriority=Speed  OutDataTypeStr=uint16  RndMeth=Nearest  InputSameDT=on
  1-D Lookup Table1 : Lookup_n-D  NumberOfTableDimensions=1  BreakpointsForDimension1=APPS2_Voltage  Table=APPS_Map  ExtrapMethod=Clip  InternalRulePriority=Speed  OutDataTypeStr=uint16  RndMeth=Nearest  InputSameDT=on
  APPS1 : ec55xxlib/RapidECU_U2/02AnalogInput/AnalogInput  channel=54: I_AN15_5V  sampletime=-1
  APPS2 : ec55xxlib/RapidECU_U2/02AnalogInput/AnalogInput  channel=55: I_AN16_5V  sampletime=-1
  "Filter1 " : Subsystem
  "Filter2 " : Subsystem
  Reliability testing : Subsystem
  SCS_Wire_breakage_detection : Subsystem
  Subsystem : Subsystem
  APPS_Pos : Outport
  APPS_Unreliable : Outport  Port=2
  APPS1_Disconnect : Outport  Port=3
  APPS2_Disconnect : Outport  Port=4
  wires:
  "Filter2 "/1(Out) -> SCS_Wire_breakage_detection/2(APPS2_Voltage), 1-D Lookup Table1/1
  APPS2/1 -> "Filter2 "/1(In)  "APPS2_Vol_In"
  "Filter1 "/1(Out) -> 1-D Lookup Table/1, SCS_Wire_breakage_detection/1(APPS1_Voltage)
  APPS1/1 -> "Filter1 "/1(In)  "APPS1_Vol_In"
  1-D Lookup Table/1 -> Reliability testing/1(APPS1_Pos), Subsystem/1(APPS1_Pos)  "APPS1_Pos"
  1-D Lookup Table1/1 -> Subsystem/2(APPS2_Pos), Reliability testing/2(APPS2_Pos)  "APPS2_Pos"
  Subsystem/1(APPS_Pos) -> APPS_Pos/1  "APPS_Pos"
  Reliability testing/1(APPS_Unreliable) -> APPS_Unreliable/1  "APPS_Unreliable"
  SCS_Wire_breakage_detection/1(APPS1_Disconnect) -> APPS1_Disconnect/1  "APPS1_Disconnect"
  SCS_Wire_breakage_detection/2(APPS2_Disconnect) -> APPS2_Disconnect/1  "APPS2_Disconnect"

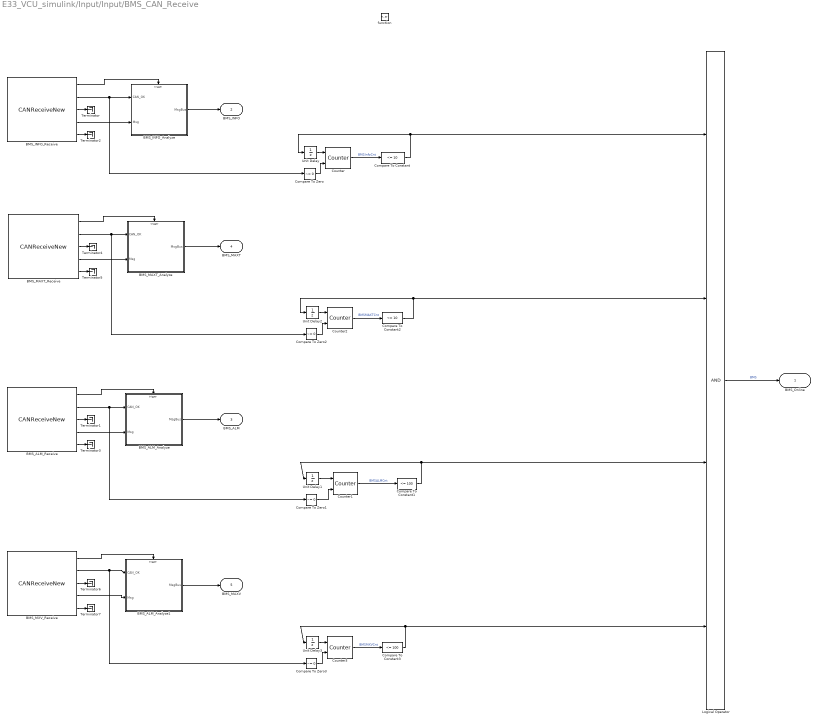
== system E33_VCU_simulink/Input/Input/BMS_CAN_Receive ==
  function : TriggerPort  TriggerType=function-call
  BMS_ALM_Analyze : Subsystem  TreatAsAtomicUnit=on
  BMS_ALM_Analyze1 : Subsystem  TreatAsAtomicUnit=on
  BMS_ALM_Receive : ec55xxlib/RapidECU_U2/07CANCommucation/CANReceiveNew  canmodule=A  canbuffer=5  canmessageid=hex2dec('186540F3')  canmessagetype=Extended(29-bit ID)  datalength=8  sampletime=-1
  BMS_INFO_Analyze : Subsystem  TreatAsAtomicUnit=on
  BMS_INFO_Receive : ec55xxlib/RapidECU_U2/07CANCommucation/CANReceiveNew  canmodule=A  canbuffer=3  canmessageid=hex2dec('186040F3')  canmessagetype=Extended(29-bit ID)  datalength=8  sampletime=-1
  BMS_MAXT_Analyze : Subsystem  TreatAsAtomicUnit=on
  BMS_MAXT_Receive : ec55xxlib/RapidECU_U2/07CANCommucation/CANReceiveNew  canmodule=A  canbuffer=4  canmessageid=hex2dec('186240F3')  canmessagetype=Extended(29-bit ID)  datalength=8  sampletime=-1
  BMS_MXV_Receive : ec55xxlib/RapidECU_U2/07CANCommucation/CANReceiveNew  canmodule=A  canbuffer=6  canmessageid=hex2dec('186140F3')  canmessagetype=Extended(29-bit ID)  datalength=8  sampletime=-1
  Compare To Constant : simulink/Logic and Bit Operations/Compare To Constant  relop=<=  const=10  OutDataTypeStr=uint8
  Compare To Constant1 : simulink/Logic and Bit Operations/Compare To Constant  relop=<=  const=100  OutDataTypeStr=uint8
  Compare To Constant2 : simulink/Logic and Bit Operations/Compare To Constant  relop=<=  const=10  OutDataTypeStr=uint8
  Compare To Constant3 : simulink/Logic and Bit Operations/Compare To Constant  relop=<=  const=100  OutDataTypeStr=uint8
  Compare To Zero{,1..3} (4 alike) : simulink/Logic and Bit Operations/Compare To Zero  relop=~=  OutDataTypeStr=boolean
  Counter{,1..3} (4 alike) : dspswit3/Counter  Direction=Up  CountEvent=Non-zero sample  CounterSize=8 bits  MaxCount=255  InitialCount=0  Output=Count  HitValue=5  ResetInput=on  SamplesPerFrame=1  Ts=-1  CntDtype=uint8  HitDtype=Logical
  Logical Operator : Logic  Inputs=4  AllPortsSameDT=off  OutDataTypeStr=boolean
  Terminator{,1..7} (8 alike) : Terminator
  Unit Delay{,1..3} (4 alike) : UnitDelay  SampleTime=-1
  BMS_Online : Outport
  BMS_INFO : Outport  Port=2
  BMS_ALM : Outport  Port=3
  BMS_MAXT : Outport  Port=4
  BMS_MAXV : Outport  Port=5
  wires:
  BMS_INFO_Receive/4 -> BMS_INFO_Analyze/2(Msg)
  BMS_INFO_Receive/5 -> Terminator2/1
  BMS_INFO_Receive/3 -> Terminator/1
  BMS_INFO_Receive/2 -> Compare To Zero/1, BMS_INFO_Analyze/1(CAN_OK)
  Compare To Constant/1 -> Unit Delay/1, Logical Operator/1
  Counter/1 -> Compare To Constant/1  "BMSInfoCnt"
  Unit Delay/1 -> Counter/1
  Compare To Zero/1 -> Counter/2
  BMS_INFO_Analyze/1(MsgBus) -> BMS_INFO/1
  BMS_INFO_Receive/1 -> BMS_INFO_Analyze/Trigger
  BMS_ALM_Receive/3 -> Terminator1/1
  BMS_ALM_Receive/5 -> Terminator3/1
  BMS_ALM_Receive/4 -> BMS_ALM_Analyze/2(Msg)
  BMS_ALM_Receive/1 -> BMS_ALM_Analyze/Trigger
  BMS_ALM_Analyze/1(MsgBus) -> BMS_ALM/1
  BMS_ALM_Receive/2 -> Compare To Zero1/1, BMS_ALM_Analyze/1(CAN_OK)
  Compare To Constant1/1 -> Unit Delay1/1, Logical Operator/3
  Counter1/1 -> Compare To Constant1/1  "BMSALMCnt"
  Unit Delay1/1 -> Counter1/1
  Compare To Zero1/1 -> Counter1/2
  Logical Operator/1 -> BMS_Online/1  "BMS"
  BMS_MAXT_Receive/3 -> Terminator4/1
  BMS_MAXT_Receive/5 -> Terminator5/1
  BMS_MAXT_Receive/4 -> BMS_MAXT_Analyze/2(Msg)
  BMS_MAXT_Receive/1 -> BMS_MAXT_Analyze/Trigger
  BMS_MAXT_Analyze/1(MsgBus) -> BMS_MAXT/1
  BMS_MAXT_Receive/2 -> BMS_MAXT_Analyze/1(CAN_OK), Compare To Zero2/1
  Compare To Constant2/1 -> Unit Delay2/1, Logical Operator/2
  Counter2/1 -> Compare To Constant2/1  "BMSMAXTCnt"
  Unit Delay2/1 -> Counter2/1
  Compare To Zero2/1 -> Counter2/2
  BMS_MXV_Receive/3 -> Terminator6/1
  BMS_MXV_Receive/5 -> Terminator7/1
  BMS_MXV_Receive/4 -> BMS_ALM_Analyze1/2(Msg)
  BMS_MXV_Receive/1 -> BMS_ALM_Analyze1/Trigger
  BMS_ALM_Analyze1/1(MsgBus) -> BMS_MAXV/1
  BMS_MXV_Receive/2 -> Compare To Zero3/1, BMS_ALM_Analyze1/1(CAN_OK)
  Compare To Constant3/1 -> Unit Delay3/1, Logical Operator/4
  Unit Delay3/1 -> Counter3/1
  Compare To Zero3/1 -> Counter3/2
  Counter3/1 -> Compare To Constant3/1  "BMSMXVCnt"

== system E33_VCU_simulink/Input/Input/Bpressure ==
  function : TriggerPort  TriggerType=function-call
  1-D Lookup Table : Lookup_n-D  NumberOfTableDimensions=1  BreakpointsForDimension1=BP_R_Voltage  Table=BP_Map  ExtrapMethod=Clip  InternalRulePriority=Speed  OutDataTypeStr=uint16  RndMeth=Simplest  InputSameDT=on
  1-D Lookup Table1 : Lookup_n-D  NumberOfTableDimensions=1  BreakpointsForDimension1=BP_F_Voltage  Table=BP_Map  ExtrapMethod=Clip  InternalRulePriority=Speed  OutDataTypeStr=uint16  RndMeth=Simplest  InputSameDT=on
  BPressure_F : ec55xxlib/RapidECU_U2/02AnalogInput/AnalogInput  channel=53: I_AN14_5V  sampletime=-1
  BPressure_R : ec55xxlib/RapidECU_U2/02AnalogInput/AnalogInput  channel=52: I_AN13_5V  sampletime=-1
  SCS_Wire_breakage_detection : Subsystem
  BP_F_Pos : Outport
  BP_R_Pos : Outport  Port=2
  BP_F_Disconnect : Outport  Port=3
  BP_R_Disconnect : Outport  Port=4
  wires:
  1-D Lookup Table1/1 -> BP_F_Pos/1  "BP_F_Pos"
  1-D Lookup Table/1 -> BP_R_Pos/1  "BP_R_Pos"
  BPressure_R/1 -> 1-D Lookup Table/1, SCS_Wire_breakage_detection/2(BP_R_Voltage)  "BP_R_Vol_In"
  BPressure_F/1 -> 1-D Lookup Table1/1, SCS_Wire_breakage_detection/1(BP_F_Voltage)  "BP_F_Vol_In"
  SCS_Wire_breakage_detection/1(BP_F_Disconnect) -> BP_F_Disconnect/1  "BP_F_Disconnect"
  SCS_Wire_breakage_detection/2(BP_R_Disconnect) -> BP_R_Disconnect/1  "BP_R_Disconnect"

== system E33_VCU_simulink/Input/Input/Keys ==
  function : TriggerPort  TriggerType=function-call
  BoolFilter6 : Subsystem
  Logical Operator : Logic  Operator=NOT  Inputs=1  AllPortsSameDT=off  OutDataTypeStr=boolean
  R2D_In : ec55xxlib/RapidECU_U2/01SwitchInput/SwitchInput  channel=6: I_SW01_L  sampletime=-1
  R2D_SW : Outport
  wires:
  R2D_In/1 -> BoolFilter6/1(Raw)
  BoolFilter6/1(Filtered) -> Logical Operator/1
  Logical Operator/1 -> R2D_SW/1

== system E33_VCU_simulink/Input/Input/MCU_CAN_Receive ==
  function : TriggerPort  TriggerType=function-call
  CANReceive : ec55xxlib/RapidECU_U2/07CANCommucation/CANReceive  canmodule=A  canbuffer=1  canmessageid=hex2dec('0CFFC6EF')  canmessagetype=Extended(29-bit ID)  datalength=8  sampletime=-1
  CANReceive1 : ec55xxlib/RapidECU_U2/07CANCommucation/CANReceive  canmodule=A  canbuffer=2  canmessageid=hex2dec('0CFFC7EF')  canmessagetype=Extended(29-bit ID)  datalength=8  sampletime=-1
  Compare To Constant1 : simulink/Logic and Bit Operations/Compare To Constant  relop=<=  const=10  OutDataTypeStr=uint8
  Compare To Constant2 : simulink/Logic and Bit Operations/Compare To Constant  relop=<=  const=10  OutDataTypeStr=uint8
  Compare To Zero : simulink/Logic and Bit Operations/Compare To Zero  relop=~=  OutDataTypeStr=boolean
  Compare To Zero1 : simulink/Logic and Bit Operations/Compare To Zero  relop=~=  OutDataTypeStr=boolean
  Counter1 : dspswit3/Counter  Direction=Up  CountEvent=Non-zero sample  CounterSize=32 bits  MaxCount=255  InitialCount=0  Output=Count  HitValue=5  ResetInput=on  SamplesPerFrame=1  Ts=-1  CntDtype=uint32  HitDtype=Logical
  Counter2 : dspswit3/Counter  Direction=Up  CountEvent=Non-zero sample  CounterSize=32 bits  MaxCount=255  InitialCount=0  Output=Count  HitValue=5  ResetInput=on  SamplesPerFrame=1  Ts=-1  CntDtype=uint32  HitDtype=Logical
  Logical Operator1 : Logic  AllPortsSameDT=off  OutDataTypeStr=boolean
  ReceiveMessages : Subsystem
  ReceiveMessages1 : Subsystem
  Terminator{,1..3} (4 alike) : Terminator
  Unit Delay1 : UnitDelay  SampleTime=-1
  Unit Delay2 : UnitDelay  SampleTime=-1
  MCU_Online : Outport
  MCU_Stat : Outport  Port=2
  MCU_Power : Outport  Port=3
  wires:
  CANReceive/5 -> Terminator1/1
  CANReceive/3 -> Terminator/1
  CANReceive/1 -> ReceiveMessages/Trigger
  CANReceive/2 -> Compare To Zero/1, ReceiveMessages/1(CAN_OK)  "Infomation_OK"
  CANReceive/4 -> ReceiveMessages/2(Msg)
  Counter1/1 -> Compare To Constant1/1  "McuInfoOfflineCnt"
  Compare To Zero/1 -> Counter1/2
  Compare To Constant1/1 -> Unit Delay1/1, Logical Operator1/1  "MCU_Stat_Online"
  Unit Delay1/1 -> Counter1/1
  CANReceive1/5 -> Terminator3/1
  CANReceive1/3 -> Terminator2/1
  CANReceive1/1 -> ReceiveMessages1/Trigger
  CANReceive1/2 -> ReceiveMessages1/1(CAN_OK), Compare To Zero1/1  "State_OK"
  CANReceive1/4 -> ReceiveMessages1/2(Msg)
  Counter2/1 -> Compare To Constant2/1  "McuStatelineCnt"
  Compare To Zero1/1 -> Counter2/2
  Compare To Constant2/1 -> Unit Delay2/1, Logical Operator1/2  "MCU_Power_Online"
  Unit Delay2/1 -> Counter2/1
  Logical Operator1/1 -> MCU_Online/1  "MCU_Online"
  ReceiveMessages/1(CAN_MCU_Stat) -> MCU_Stat/1
  ReceiveMessages1/1(CAN_MCU_Pwr) -> MCU_Power/1

== system E33_VCU_simulink/Input/Input/Self_inspection ==
  function : TriggerPort  TriggerType=function-call
  APPS1_PWR : ec55xxlib/RapidECU_U2/09PowerManagement/PowerVoltageMonitor  channel=80: O_5V1_100MA  sampletime=-1
  APPS2_PWR : ec55xxlib/RapidECU_U2/09PowerManagement/PowerVoltageMonitor  channel=81: O_5V2_50MA  sampletime=-1
  BP_PWR : ec55xxlib/RapidECU_U2/09PowerManagement/PowerVoltageMonitor  channel=76: O_AP1_300MA  sampletime=-1
  I_BAT : ec55xxlib/RapidECU_U2/09PowerManagement/PowerVoltageMonitor  channel=4: I_BAT  sampletime=-1
  I_UBR : ec55xxlib/RapidECU_U2/09PowerManagement/PowerVoltageMonitor  channel=116: I_UBR  sampletime=-1
  PWR_5V : ec55xxlib/RapidECU_U2/09PowerManagement/PowerVoltageMonitor  channel=76: O_AP1_300MA  sampletime=-1
  Terminator{,1..5} (6 alike) : Terminator
  wires:
  I_UBR/1 -> Terminator1/1  "I_UBR"
  BP_PWR/1 -> Terminator2/1  "BP_PWR"
  APPS1_PWR/1 -> Terminator3/1  "APPS1_PWR"
  APPS2_PWR/1 -> Terminator4/1  "APPS2_PWR"
  PWR_5V/1 -> Terminator5/1  "PWR_5V"
  I_BAT/1 -> Terminator/1  "I_BAT"
